simulink model "sim_ai_smc"  (R2023b)
settings: Solver=ode1  StartTime=0.0  StopTime=2  FixedStep=0.0001  RelTol=1e-3
values from neighbouring files (symbols this model uses):
  Te = 0.001    [ai_smc.m]    (also in fsmc.m; ismc.m; st_smc.m)
  Tm = 0.2    [ai_smc.m]    (also in fsmc.m; ismc.m; st_smc.m)
  ts = 1e-4    (= 0.0001)    [ai_smc.m]    (also in fsmc.m; ismc.m; st_smc.m)
libraries: fuzblock x1
settings Model: Creator=HP  LastModifiedBy=HP

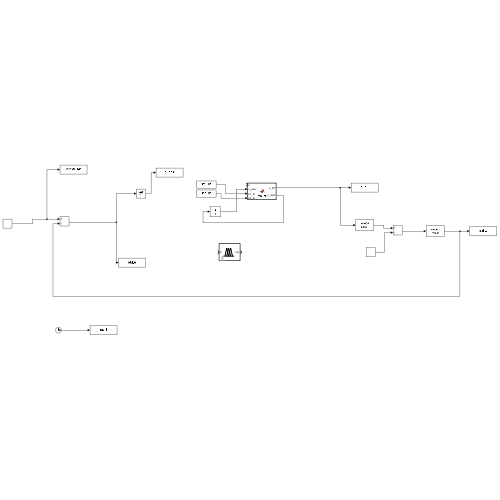
[thumbnail: Simulink's stored preview of the top-level diagram]
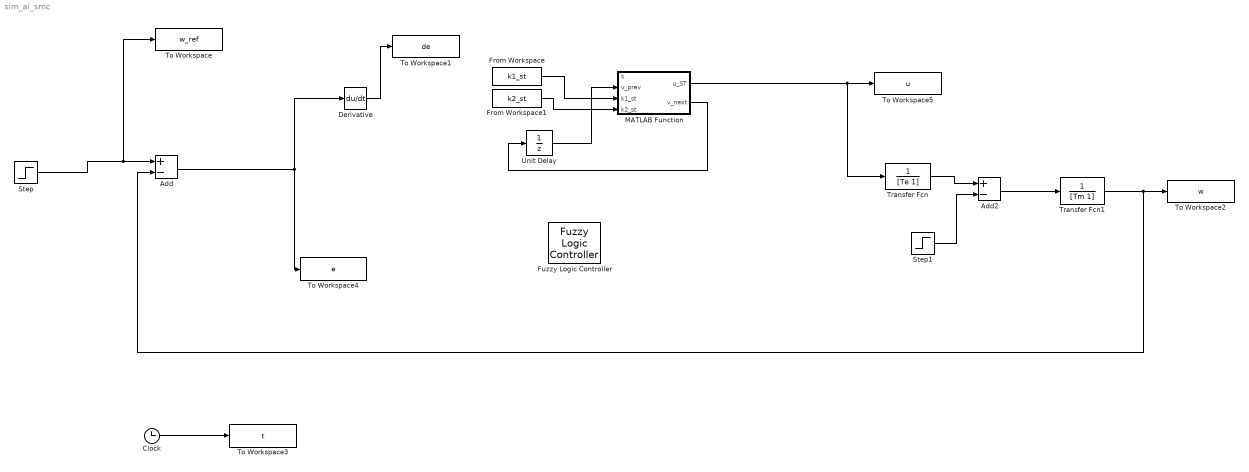
== system sim_ai_smc ==
  Add : Sum  Inputs=+-
  Add2 : Sum  Inputs=+-
  Clock : Clock
  Derivative : Derivative
  From Workspace : FromWorkspace  VariableName=k1_st
  From Workspace1 : FromWorkspace  VariableName=k2_st
  Fuzzy Logic Controller : fuzblock/Fuzzy Logic  Controller  FIS=ai_smc_fuzzy  OutputSampleNumber=101  DataType=double  FuzzifiedInputs=off  RuleFiringStrengths=off  RuleOutputs=off  AggregatedOutputs=off  SimulateUsing=Interpreted execution  OutOfRangeInputValueMessage=warning  NoRuleFiredMessage=warning  EmptyOutputFuzzySetMessage=warning
  MATLAB Function : MATLAB Function  TreatAsAtomicUnit=on
  Step : Step  Time=0.1  SampleTime=0
  Step1 : Step  SampleTime=0
  To Workspace : ToWorkspace  VariableName=w_ref  SaveFormat=Timeseries  SampleTime=-1
  To Workspace1 : ToWorkspace  VariableName=de  SaveFormat=Timeseries  SampleTime=-1
  To Workspace2 : ToWorkspace  VariableName=w  SaveFormat=Timeseries  SampleTime=-1
  To Workspace3 : ToWorkspace  VariableName=t  SaveFormat=Timeseries  SampleTime=-1
  To Workspace4 : ToWorkspace  VariableName=e  SaveFormat=Timeseries  SampleTime=-1
  To Workspace5 : ToWorkspace  VariableName=u  SaveFormat=Timeseries  SampleTime=-1
  Transfer Fcn : TransferFcn  Denominator=[Te 1]
  Transfer Fcn1 : TransferFcn  Denominator=[Tm 1]
  Unit Delay : UnitDelay  SampleTime=ts  HasFrameUpgradeWarning=on
  wires:
  Clock/1 -> To Workspace3/1
  Transfer Fcn1/1 -> Add/2, To Workspace2/1
  Step1/1 -> Add2/2
  Add2/1 -> Transfer Fcn1/1
  Transfer Fcn/1 -> Add2/1
  Derivative/1 -> To Workspace1/1
  Unit Delay/1 -> MATLAB Function/2(v_prev)
  Step/1 -> To Workspace/1, Add/1
  MATLAB Function/1(u_ST) -> Transfer Fcn/1, To Workspace5/1
  MATLAB Function/2(v_next) -> Unit Delay/1
  Add/1 -> Derivative/1, To Workspace4/1
  From Workspace/1 -> MATLAB Function/3(k1_st)
  From Workspace1/1 -> MATLAB Function/4(k2_st)

== matlab function sim_ai_smc/MATLAB Function ==
  data: s input; u_ST output; v_prev input; v_next output; k1_st input; k2_st input
function [u_ST, v_next] = fcn_st(s, v_prev, k1_st, k2_st)
% Bazowa składowa Super-Twisting SMC (u_ST)
% Adaptacyjna korekcja u_fuzzy jest dodawana w Simulinku

ts = 1e-4;     % Krok czasowy
eps = 1e-3;    % Strefa martwa dla znaku
eps2 = 1e-12;  % Zapobieganie dzieleniu przez zero

% 1) przybliżony sign
sign_approx = max(-1, min(1, s/eps));

% 2) dyskretna integracja v
v_next = v_prev + ts * sign_approx;

% 3) składowa pierwiastkowa (u1)
u1 = k1_st * sqrt(abs(s) + eps2) * sign_approx;

% 4) składowa zależna od v (u2)
u2 = k2_st * v_next;

% 5) suma bazowego sterowania ST-SMC (BEZ saturacji, ponieważ saturacja
% powinna być na końcu, po dodaniu u_fuzzy)
u_ST = u1 + u2;

end
